simulink model "model_1Vexp2V_SexpS"  (R2023a)
settings: Solver=VariableStepAuto  StartTime=0.0  StopTime=length(data)/100  RelTol=1e-3
values from neighbouring files (symbols this model uses):
  a = A(3)    [F1Vexp2V.m]    (also in F1Vexp2V_SexpS.m; F1Vexp2V_SexpS_ssr_all.m = input_parameters(3); F1Vexp3V.m; F1VexpV.m)
  b = A(3)    [F1Sy.m]    (also in F1Vexp2V_SexpS.m = A(4); F1Vexp2V_SexpS_ssr.m = abs(b); F1Vexp2V_SexpS_ssr_all.m = input_parameters(5); F1VxSy.m = A(4))
  data = load(input_data)    [F1.m]    (also in F1Sy.m; F1Vexp2V.m; F1Vexp2V_SexpS.m; F1Vexp2V_SexpS_ssr.m)
  R = A(2)    [F1.m]    (also in F1Sy.m; F1Vexp2V.m; F1Vexp2V_SexpS.m; F1Vexp2V_SexpS_ssr_all.m = input_parameters(2))
  x = input_parameters(1)    [F1Vexp2V_SexpS_ssr.m]    (also in F1Vexp2V_SexpS_ssr_all.m = input_parameters(4); F1Vexp2V_ssr.m; F1Vexp3V_ssr.m; F1VexpV_ssr.m)
  y = input_parameters(2)    [F1Vexp2V_SexpS_ssr.m]    (also in F1Vexp2V_SexpS_ssr_all.m = input_parameters(6))
settings Model: Creator=test  LastModifiedBy=test
settings DebuggingCC: AlgebraicLoopMsg=none

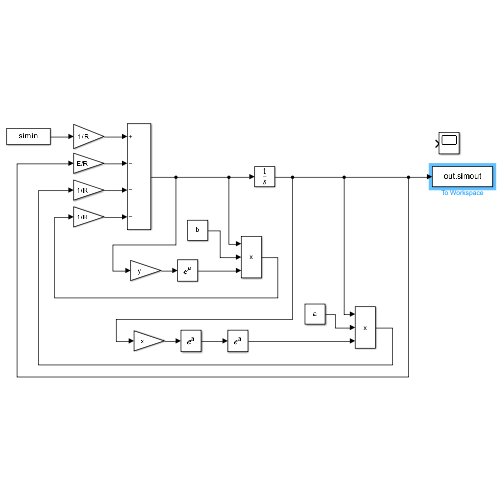
[thumbnail: Simulink's stored preview of the top-level diagram]
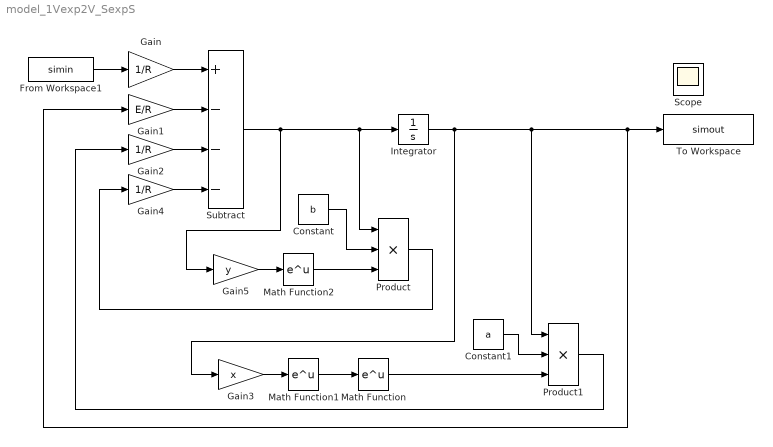
== system model_1Vexp2V_SexpS ==
  Constant : Constant  Value=b
  Constant1 : Constant  Value=a
  From Workspace1 : FromWorkspace  VariableName=simin
  Gain : Gain  Gain=1/R
  Gain1 : Gain  Gain=E/R
  Gain2 : Gain  Gain=1/R
  Gain3 : Gain  Gain=x
  Gain4 : Gain  Gain=1/R
  Gain5 : Gain  Gain=y
  Integrator : Integrator  InitialCondition=data(1,3)
  Math Function : Math
  Math Function1 : Math
  Math Function2 : Math
  Product : Product  Inputs=3
  Product1 : Product  Inputs=3
  Scope : Scope
  Subtract : Sum  Inputs=+---
  To Workspace : ToWorkspace  VariableName=simout  SaveFormat=Timeseries  SampleTime=0.01
  wires:
  Gain1/1 -> Subtract/2
  Gain2/1 -> Subtract/3
  From Workspace1/1 -> Gain/1
  Gain/1 -> Subtract/1
  Integrator/1 -> To Workspace/1, Gain1/1, Product1/1, Gain3/1
  Gain3/1 -> Math Function1/1
  Math Function1/1 -> Math Function/1
  Gain4/1 -> Subtract/4
  Subtract/1 -> Product/1, Integrator/1, Gain5/1
  Gain5/1 -> Math Function2/1
  Math Function2/1 -> Product/3
  Constant/1 -> Product/2
  Product/1 -> Gain4/1
  Math Function/1 -> Product1/3
  Product1/1 -> Gain2/1
  Constant1/1 -> Product1/2
